simulink model "UiRlab5_model"  (R2021a)
settings: Solver=VariableStepAuto  StartTime=0.0  StopTime=tsim  RelTol=1e-3
undefined symbols (not defined in the file): Ian, K, Ka, Ki, Kria, Krib, Kt, Ktr, Kzi, Ta, Ti, Tii, Tt, Ttr, Tzi
settings Model: Creator=Luka  LastModifiedBy=Luka

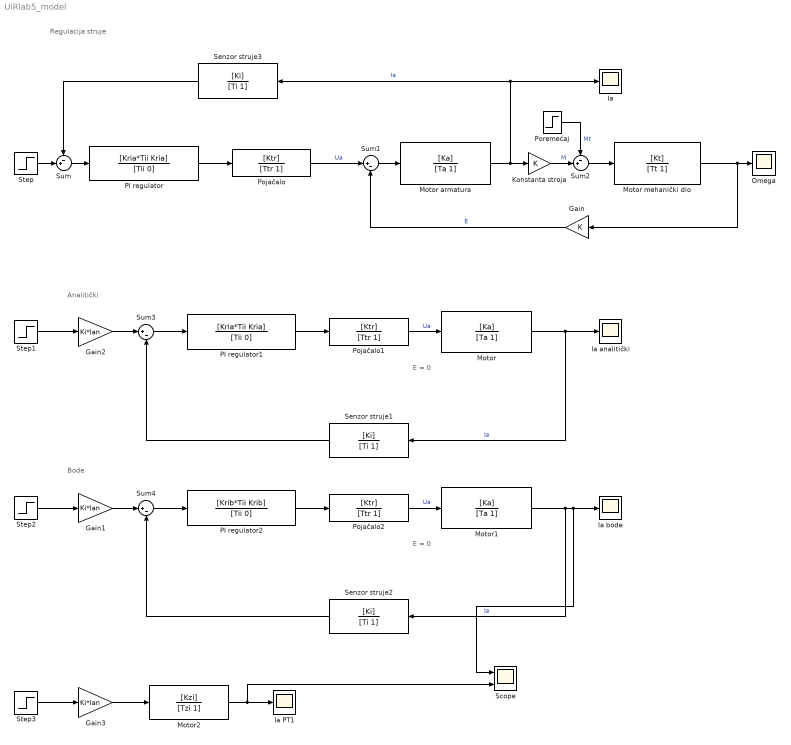
== system UiRlab5_model ==
  note: Analitički
  note: Regulacija struje
  note: E = 0
  note: E = 0
  note: Bode
  Gain : Gain  Gain=K
  Gain1 : Gain  Gain=Ki*Ian
  Gain2 : Gain  Gain=Ki*Ian
  Gain3 : Gain  Gain=Ki*Ian
  Ia : Scope
  Ia PT1 : Scope
  Ia analitički : Scope
  Ia bode : Scope
  Konstanta stroja : Gain  Gain=K
  "Motor " : TransferFcn  Numerator=[Ka]  Denominator=[Ta 1]
  Motor armatura : TransferFcn  Numerator=[Ka]  Denominator=[Ta 1]
  Motor mehanički dio : TransferFcn  Numerator=[Kt]  Denominator=[Tt 1]
  Motor1 : TransferFcn  Numerator=[Ka]  Denominator=[Ta 1]
  Motor2 : TransferFcn  Numerator=[Kzi]  Denominator=[Tzi 1]
  Omega : Scope
  PI regulator : TransferFcn  Numerator=[Kria*Tii Kria]  Denominator=[Tii 0]
  PI regulator1 : TransferFcn  Numerator=[Kria*Tii Kria]  Denominator=[Tii 0]
  PI regulator2 : TransferFcn  Numerator=[Krib*Tii Krib]  Denominator=[Tii 0]
  Pojačalo : TransferFcn  Numerator=[Ktr]  Denominator=[Ttr 1]
  Pojačalo1 : TransferFcn  Numerator=[Ktr]  Denominator=[Ttr 1]
  Pojačalo2 : TransferFcn  Numerator=[Ktr]  Denominator=[Ttr 1]
  Poremećaj : Step  Time=0  After=0  SampleTime=0
  Scope : Scope  NumInputPorts=2
  Senzor struje1 : TransferFcn  Numerator=[Ki]  Denominator=[Ti 1]
  Senzor struje2 : TransferFcn  Numerator=[Ki]  Denominator=[Ti 1]
  Senzor struje3 : TransferFcn  Numerator=[Ki]  Denominator=[Ti 1]
  Step : Step  Time=0  After=Ki*Ian  SampleTime=0
  Step1 : Step  Time=0  SampleTime=0
  Step2 : Step  Time=0  SampleTime=0
  Step3 : Step  Time=0  SampleTime=0
  Sum : Sum  Inputs=-+|
  Sum1 : Sum  Inputs=|+-
  Sum2 : Sum  Inputs=-+|
  Sum3 : Sum  Inputs=|+-
  Sum4 : Sum  Inputs=|+-
  wires:
  Step/1 -> Sum/2
  Sum/1 -> PI regulator/1
  PI regulator/1 -> Pojačalo/1
  Senzor struje3/1 -> Sum/1
  Pojačalo/1 -> Sum1/1  "Ua"
  Gain/1 -> Sum1/2  "E"
  Sum1/1 -> Motor armatura/1
  Motor armatura/1 -> Senzor struje3/1, Ia/1, Konstanta stroja/1  "Ia"
  Konstanta stroja/1 -> Sum2/2  "M"
  Poremećaj/1 -> Sum2/1  "Mt"
  Motor mehanički dio/1 -> Gain/1, Omega/1
  Sum2/1 -> Motor mehanički dio/1
  Step1/1 -> Gain2/1
  Gain2/1 -> Sum3/1
  Sum3/1 -> PI regulator1/1
  PI regulator1/1 -> Pojačalo1/1
  Pojačalo1/1 -> "Motor "/1  "Ua"
  "Motor "/1 -> Senzor struje1/1, Ia analitički/1  "Ia"
  Senzor struje1/1 -> Sum3/2
  Senzor struje2/1 -> Sum4/2
  Motor1/1 -> Scope/1, Ia bode/1, Senzor struje2/1  "Ia"
  Pojačalo2/1 -> Motor1/1  "Ua"
  PI regulator2/1 -> Pojačalo2/1
  Sum4/1 -> PI regulator2/1
  Gain1/1 -> Sum4/1
  Step2/1 -> Gain1/1
  Step3/1 -> Gain3/1
  Gain3/1 -> Motor2/1
  Motor2/1 -> Scope/2, Ia PT1/1
